simulink model "floribot_wiimote"  (R2013a)
settings: Solver=FixedStepDiscrete  StartTime=0.0  StopTime=inf  RelTol=1e-3  SampleTimeConstraint=STIndependent
settings Model: Creator=Torsten  LastModifiedBy=Torsten
settings OptimizationCC: OptimizeModelRefInitCode=on  LifeSpan=Inf
settings RTWCC: SystemTargetFile=ert.tlc  GenCodeOnly=on  GenerateMakefile=off  TemplateMakefile=ert_default_tmf  Description=Embedded Coder  ProcessScript=ert_make_rtw_hook  TargetLang=C++
settings CodeAppCC: IgnoreCustomStorageClasses=off
settings ERTTargetCC: InlinedParameterPlacement=Hierarchical  ERTCustomFileTemplate=example_file_process.tlc

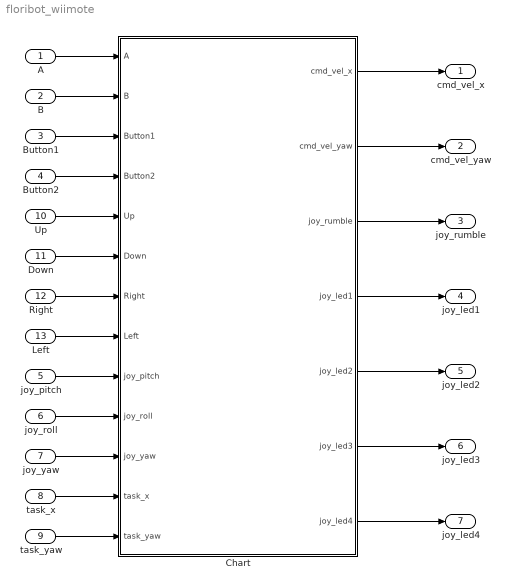
== system floribot_wiimote ==
  A : Inport
  B : Inport  Port=2
  Button1 : Inport  Port=3
  Button2 : Inport  Port=4
  joy_pitch : Inport  Port=5
  joy_roll : Inport  Port=6
  joy_yaw : Inport  Port=7
  task_x : Inport  Port=8
  task_yaw : Inport  Port=9
  Up : Inport  Port=10
  Down : Inport  Port=11
  Right : Inport  Port=12
  Left : Inport  Port=13
  Chart : Stateflow chart  TreatAsAtomicUnit=on
  cmd_vel_x : Outport
  cmd_vel_yaw : Outport  Port=2
  joy_rumble : Outport  Port=3
  joy_led1 : Outport  Port=4
  joy_led2 : Outport  Port=5
  joy_led3 : Outport  Port=6
  joy_led4 : Outport  Port=7
  wires:
  A/1 -> Chart/1(A)
  B/1 -> Chart/2(B)
  Button1/1 -> Chart/3(Button1)
  Button2/1 -> Chart/4(Button2)
  joy_pitch/1 -> Chart/9(joy_pitch)
  joy_yaw/1 -> Chart/11(joy_yaw)
  joy_roll/1 -> Chart/10(joy_roll)
  task_x/1 -> Chart/12(task_x)
  task_yaw/1 -> Chart/13(task_yaw)
  Chart/1(cmd_vel_x) -> cmd_vel_x/1
  Chart/2(cmd_vel_yaw) -> cmd_vel_yaw/1
  Chart/3(joy_rumble) -> joy_rumble/1
  Chart/4(joy_led1) -> joy_led1/1
  Chart/7(joy_led4) -> joy_led4/1
  Chart/6(joy_led3) -> joy_led3/1
  Chart/5(joy_led2) -> joy_led2/1
  Up/1 -> Chart/5(Up)
  Down/1 -> Chart/6(Down)
  Right/1 -> Chart/7(Right)
  Left/1 -> Chart/8(Left)

== stateflow chart floribot_wiimote/Chart ==
  state manual
    joy_led1 = true;
    joy_led2 = false;
    joy_led3 = false;
    joy_led4 = false;
    state stand_still
      cmd_vel_x = 0;
      cmd_vel_yaw = 0;
    state control_x_and_yaw
      during:
      cmd_vel_x = joy_pitch/DIRECT_PITCH_AXIS_DIV;
      cmd_vel_yaw = joy_roll/DIRECT_ROLL_AXIS_DIV;
    state Up
    state Down
    state Right
    state Left
    (default) -> stand_still
    stand_still -> control_x_and_yaw [order 1] : [B]
    control_x_and_yaw -> stand_still : [!B]
    Up -> Up [order 2] : [joy_pitch > 0]/cmd_vel_x = joy_pitch/DIRECT_PITCH_AXIS_DIV;
    stand_still -> Up [order 2] : [Up]
    Up -> stand_still [order 1] : [!Up]
    stand_still -> Down [order 3] : [Down]
    Down -> Down [order 2] : [joy_pitch < 0]/cmd_vel_x = joy_pitch/DIRECT_PITCH_AXIS_DIV;
    Down -> stand_still [order 1] : [!Down]
    stand_still -> Right [order 4] : [Right]
    Right -> Right [order 2] : [joy_roll > 0]/cmd_vel_yaw = joy_roll/DIRECT_ROLL_AXIS_DIV;
    Right -> stand_still [order 1] : [!Right]
    Left -> Left [order 2] : [joy_roll < 0]/cmd_vel_yaw = joy_roll/DIRECT_ROLL_AXIS_DIV;
    stand_still -> Left [order 5] : [Left]
    Left -> stand_still [order 1] : [!Left]
  state automatic
    during:
    cmd_vel_x = task_x;
    cmd_vel_yaw = task_yaw;
    joy_led1 = false;
    joy_led2 = true;
    joy_led3 = false;
    joy_led4 = false;
  (default) -> manual
  automatic -> manual : [Button1]
  manual -> automatic : [Button2 && !Button1]
  data: A input boolean; B input boolean; Button1 input boolean; Button2 input boolean; Up input boolean; Down input boolean; Right input boolean; Left input boolean; joy_pitch input double; joy_roll input double; joy_yaw input double; task_x input double; task_yaw input double; cmd_vel_x output double; cmd_vel_yaw output double; joy_rumble output double; joy_led1 output boolean; joy_led2 output boolean; joy_led3 output boolean; joy_led4 output boolean; DIRECT_PITCH_AXIS_DIV constant double =10; DIRECT_ROLL_AXIS_DIV constant double =-30
